simulink model "Basic_DMT"  (R2014b)
settings: Solver=FixedStepDiscrete  SolverMode=SingleTasking  StartTime=0.0  StopTime=25e-6-14e-9*24  RelTol=1e-3
PreLoadFcn:
  | userName = getenv('UserName');
  | 
  | if strcmp(userName,'Tim')
  | cd C:\Users\Tim\Documents\GitHub\MA_1\Basic_DMT
  | else
  | cd C:\Users\Tim-UML\Documents\GitHub\MA_1\Basic_DMT
  | end
InitFcn:
  | userName = getenv('UserName');
  | 
  | if strcmp(userName,'Tim')
  | cd C:\Users\Tim\Documents\GitHub\MA_1\Basic_DMT
  | else
  | cd C:\Users\Tim-UML\Documents\GitHub\MA_1\Basic_DMT
  | end
values from neighbouring files (symbols this model uses):
  a0 = 0.21194908595403703    (= 0.211949085954)    [initScript.m]
  a1 = 0.576101828091926    (= 0.576101828092)    [initScript.m]
  a2 = a0    (= 0.211949085954)    [initScript.m]
  beta = 1    [initScript.m]
  bitPerSymb = 4    [initScript.m]
  chanDownFact = Tchan/SystemPeriod    [initScript.m]
  fftLen = 16    [initScript.m]
  fftLenActive = fftLenDMT    (= 32)    [initScript.m]
  fftLenDMT = 2*fftLen    (= 32)    [initScript.m]
  GI_Active = GI_LenDMT    (= 0)    [initScript.m]
  GI_Len = 0    [initScript.m]
  GI_LenDMT = 0    [initScript.m]
  M = log2(fftLen)    [initScript.m]
  sysgenSystemPeriod = 4e-9    (= 4e-09)    [initScript.m]
  SystemPeriod = 4e-9    (= 4e-09)    [initScript.m]
  upsampleFactor = 1    [initScript.m]
  usedSubCar = 14    [initScript.m]
undefined symbols (not defined in the file or in its folder): bitCount, get, modu_mode, Tb, Ts
libraries: xbsIndex_r4 x822, commdigbbndam3 x59, simulink x42, dspsigops x7, commrandsrc2 x6, dspbuff3 x4, dspxfrm3 x3, dspswit3 x2, commseqgen2 x1, dsparch4 x1, commutil2 x1, dspsnks4 x1
(part 6 of 10)

== system Basic_DMT/Sysgen_Modulation/16-QAM4 ==
  In1 : Inport
  BitBasher : xbsIndex_r4/BitBasher  bitexpr=|  display_expr=on  sr_1=b  arith_type1=Unsigned  bin_pt1=0  sr_2=c  arith_type2=Unsigned  bin_pt2=0  sr_3=3  arith_type3=Unsigned  bin_pt3=0  sr_4=4  arith_type4=Unsigned  bin_pt4=0  dbl_ovrd=off  block_type=bitbasher
      | b={a[3:2]}
      | c={a[1:0]}
  Constant1 : xbsIndex_r4/Constant  const=-3  gui_display_data_type=Fixed-point  arith_type=Signed (2's comp)  n_bits=bitCount  bin_pt=fracLen  preci_type=Single  exp_width=8  frac_width=24  explicit_period=on  period=Ts*usedSubCar* bitPerSymb  equ=P=C  opselect=C  inp2=PCIN>>17  opr=+  inp1=P  carry=CIN  dbl_ovrd=off  block_type=constant
  Constant2 : xbsIndex_r4/Constant  const=-1  gui_display_data_type=Fixed-point  arith_type=Signed (2's comp)  n_bits=bitCount  bin_pt=fracLen  preci_type=Single  exp_width=8  frac_width=24  explicit_period=on  period=Ts*usedSubCar* bitPerSymb  equ=P=C  opselect=C  inp2=PCIN>>17  opr=+  inp1=P  carry=CIN  dbl_ovrd=off  block_type=constant
  Constant3 : xbsIndex_r4/Constant  const=3  gui_display_data_type=Fixed-point  arith_type=Signed (2's comp)  n_bits=bitCount  bin_pt=fracLen  preci_type=Single  exp_width=8  frac_width=24  explicit_period=on  period=Ts*usedSubCar* bitPerSymb  equ=P=C  opselect=C  inp2=PCIN>>17  opr=+  inp1=P  carry=CIN  dbl_ovrd=off  block_type=constant
  Constant4 : xbsIndex_r4/Constant  const=1  gui_display_data_type=Fixed-point  arith_type=Signed (2's comp)  n_bits=bitCount  bin_pt=fracLen  preci_type=Single  exp_width=8  frac_width=24  explicit_period=on  period=Ts*usedSubCar* bitPerSymb  equ=P=C  opselect=C  inp2=PCIN>>17  opr=+  inp1=P  carry=CIN  dbl_ovrd=off  block_type=constant
  Constant5 : xbsIndex_r4/Constant  const=1  gui_display_data_type=Fixed-point  arith_type=Signed (2's comp)  n_bits=bitCount  bin_pt=fracLen  preci_type=Single  exp_width=8  frac_width=24  explicit_period=on  period=Ts*usedSubCar* bitPerSymb  equ=P=C  opselect=C  inp2=PCIN>>17  opr=+  inp1=P  carry=CIN  dbl_ovrd=off  block_type=constant
  Constant6 : xbsIndex_r4/Constant  const=-3  gui_display_data_type=Fixed-point  arith_type=Signed (2's comp)  n_bits=bitCount  bin_pt=fracLen  preci_type=Single  exp_width=8  frac_width=24  explicit_period=on  period=Ts*usedSubCar* bitPerSymb  equ=P=C  opselect=C  inp2=PCIN>>17  opr=+  inp1=P  carry=CIN  dbl_ovrd=off  block_type=constant
  Constant7 : xbsIndex_r4/Constant  const=-1  gui_display_data_type=Fixed-point  arith_type=Signed (2's comp)  n_bits=bitCount  bin_pt=fracLen  preci_type=Single  exp_width=8  frac_width=24  explicit_period=on  period=Ts*usedSubCar* bitPerSymb  equ=P=C  opselect=C  inp2=PCIN>>17  opr=+  inp1=P  carry=CIN  dbl_ovrd=off  block_type=constant
  Constant9 : xbsIndex_r4/Constant  const=3  gui_display_data_type=Fixed-point  arith_type=Signed (2's comp)  n_bits=bitCount  bin_pt=fracLen  preci_type=Single  exp_width=8  frac_width=24  explicit_period=on  period=Ts*usedSubCar* bitPerSymb  equ=P=C  opselect=C  inp2=PCIN>>17  opr=+  inp1=P  carry=CIN  dbl_ovrd=off  block_type=constant
  Mux : xbsIndex_r4/Mux  inputs=4  en=off  latency=1  precision=Full  arith_type=Unsigned  n_bits=16  bin_pt=14  quantization=Truncate  overflow=Wrap  dbl_ovrd=off  block_type=mux
  Mux1 : xbsIndex_r4/Mux  inputs=4  en=off  latency=1  precision=Full  arith_type=Unsigned  n_bits=16  bin_pt=14  quantization=Truncate  overflow=Wrap  dbl_ovrd=off  block_type=mux
  Out2 : Outport
  Out3 : Outport  Port=2
  wires:
  Mux1/1 -> Out3/1
  In1/1 -> BitBasher/1
  Constant1/1 -> Mux/2
  Constant2/1 -> Mux/3
  BitBasher/1 -> Mux/1
  Constant9/1 -> Mux1/2
  Constant5/1 -> Mux1/3
  Constant7/1 -> Mux1/5
  Constant6/1 -> Mux1/4
  BitBasher/2 -> Mux1/1
  Constant4/1 -> Mux/5
  Mux/1 -> Out2/1
  Constant3/1 -> Mux/4

== system Basic_DMT/Sysgen_Modulation/16-QAM5 ==
  In1 : Inport
  BitBasher : xbsIndex_r4/BitBasher  bitexpr=|  display_expr=on  sr_1=b  arith_type1=Unsigned  bin_pt1=0  sr_2=c  arith_type2=Unsigned  bin_pt2=0  sr_3=3  arith_type3=Unsigned  bin_pt3=0  sr_4=4  arith_type4=Unsigned  bin_pt4=0  dbl_ovrd=off  block_type=bitbasher
      | b={a[3:2]}
      | c={a[1:0]}
  Constant1 : xbsIndex_r4/Constant  const=-3  gui_display_data_type=Fixed-point  arith_type=Signed (2's comp)  n_bits=bitCount  bin_pt=fracLen  preci_type=Single  exp_width=8  frac_width=24  explicit_period=on  period=Ts*usedSubCar* bitPerSymb  equ=P=C  opselect=C  inp2=PCIN>>17  opr=+  inp1=P  carry=CIN  dbl_ovrd=off  block_type=constant
  Constant2 : xbsIndex_r4/Constant  const=-1  gui_display_data_type=Fixed-point  arith_type=Signed (2's comp)  n_bits=bitCount  bin_pt=fracLen  preci_type=Single  exp_width=8  frac_width=24  explicit_period=on  period=Ts*usedSubCar* bitPerSymb  equ=P=C  opselect=C  inp2=PCIN>>17  opr=+  inp1=P  carry=CIN  dbl_ovrd=off  block_type=constant
  Constant3 : xbsIndex_r4/Constant  const=3  gui_display_data_type=Fixed-point  arith_type=Signed (2's comp)  n_bits=bitCount  bin_pt=fracLen  preci_type=Single  exp_width=8  frac_width=24  explicit_period=on  period=Ts*usedSubCar* bitPerSymb  equ=P=C  opselect=C  inp2=PCIN>>17  opr=+  inp1=P  carry=CIN  dbl_ovrd=off  block_type=constant
  Constant4 : xbsIndex_r4/Constant  const=1  gui_display_data_type=Fixed-point  arith_type=Signed (2's comp)  n_bits=bitCount  bin_pt=fracLen  preci_type=Single  exp_width=8  frac_width=24  explicit_period=on  period=Ts*usedSubCar* bitPerSymb  equ=P=C  opselect=C  inp2=PCIN>>17  opr=+  inp1=P  carry=CIN  dbl_ovrd=off  block_type=constant
  Constant5 : xbsIndex_r4/Constant  const=1  gui_display_data_type=Fixed-point  arith_type=Signed (2's comp)  n_bits=bitCount  bin_pt=fracLen  preci_type=Single  exp_width=8  frac_width=24  explicit_period=on  period=Ts*usedSubCar* bitPerSymb  equ=P=C  opselect=C  inp2=PCIN>>17  opr=+  inp1=P  carry=CIN  dbl_ovrd=off  block_type=constant
  Constant6 : xbsIndex_r4/Constant  const=-3  gui_display_data_type=Fixed-point  arith_type=Signed (2's comp)  n_bits=bitCount  bin_pt=fracLen  preci_type=Single  exp_width=8  frac_width=24  explicit_period=on  period=Ts*usedSubCar* bitPerSymb  equ=P=C  opselect=C  inp2=PCIN>>17  opr=+  inp1=P  carry=CIN  dbl_ovrd=off  block_type=constant
  Constant7 : xbsIndex_r4/Constant  const=-1  gui_display_data_type=Fixed-point  arith_type=Signed (2's comp)  n_bits=bitCount  bin_pt=fracLen  preci_type=Single  exp_width=8  frac_width=24  explicit_period=on  period=Ts*usedSubCar* bitPerSymb  equ=P=C  opselect=C  inp2=PCIN>>17  opr=+  inp1=P  carry=CIN  dbl_ovrd=off  block_type=constant
  Constant9 : xbsIndex_r4/Constant  const=3  gui_display_data_type=Fixed-point  arith_type=Signed (2's comp)  n_bits=bitCount  bin_pt=fracLen  preci_type=Single  exp_width=8  frac_width=24  explicit_period=on  period=Ts*usedSubCar* bitPerSymb  equ=P=C  opselect=C  inp2=PCIN>>17  opr=+  inp1=P  carry=CIN  dbl_ovrd=off  block_type=constant
  Mux : xbsIndex_r4/Mux  inputs=4  en=off  latency=1  precision=Full  arith_type=Unsigned  n_bits=16  bin_pt=14  quantization=Truncate  overflow=Wrap  dbl_ovrd=off  block_type=mux
  Mux1 : xbsIndex_r4/Mux  inputs=4  en=off  latency=1  precision=Full  arith_type=Unsigned  n_bits=16  bin_pt=14  quantization=Truncate  overflow=Wrap  dbl_ovrd=off  block_type=mux
  Out2 : Outport
  Out3 : Outport  Port=2
  wires:
  Mux1/1 -> Out3/1
  In1/1 -> BitBasher/1
  Constant1/1 -> Mux/2
  Constant2/1 -> Mux/3
  BitBasher/1 -> Mux/1
  Constant9/1 -> Mux1/2
  Constant5/1 -> Mux1/3
  Constant7/1 -> Mux1/5
  Constant6/1 -> Mux1/4
  BitBasher/2 -> Mux1/1
  Constant4/1 -> Mux/5
  Mux/1 -> Out2/1
  Constant3/1 -> Mux/4

== system Basic_DMT/Sysgen_Modulation/16-QAM6 ==
  In1 : Inport
  BitBasher : xbsIndex_r4/BitBasher  bitexpr=|  display_expr=on  sr_1=b  arith_type1=Unsigned  bin_pt1=0  sr_2=c  arith_type2=Unsigned  bin_pt2=0  sr_3=3  arith_type3=Unsigned  bin_pt3=0  sr_4=4  arith_type4=Unsigned  bin_pt4=0  dbl_ovrd=off  block_type=bitbasher
      | b={a[3:2]}
      | c={a[1:0]}
  Constant1 : xbsIndex_r4/Constant  const=-3  gui_display_data_type=Fixed-point  arith_type=Signed (2's comp)  n_bits=bitCount  bin_pt=fracLen  preci_type=Single  exp_width=8  frac_width=24  explicit_period=on  period=Ts*usedSubCar* bitPerSymb  equ=P=C  opselect=C  inp2=PCIN>>17  opr=+  inp1=P  carry=CIN  dbl_ovrd=off  block_type=constant
  Constant2 : xbsIndex_r4/Constant  const=-1  gui_display_data_type=Fixed-point  arith_type=Signed (2's comp)  n_bits=bitCount  bin_pt=fracLen  preci_type=Single  exp_width=8  frac_width=24  explicit_period=on  period=Ts*usedSubCar* bitPerSymb  equ=P=C  opselect=C  inp2=PCIN>>17  opr=+  inp1=P  carry=CIN  dbl_ovrd=off  block_type=constant
  Constant3 : xbsIndex_r4/Constant  const=3  gui_display_data_type=Fixed-point  arith_type=Signed (2's comp)  n_bits=bitCount  bin_pt=fracLen  preci_type=Single  exp_width=8  frac_width=24  explicit_period=on  period=Ts*usedSubCar* bitPerSymb  equ=P=C  opselect=C  inp2=PCIN>>17  opr=+  inp1=P  carry=CIN  dbl_ovrd=off  block_type=constant
  Constant4 : xbsIndex_r4/Constant  const=1  gui_display_data_type=Fixed-point  arith_type=Signed (2's comp)  n_bits=bitCount  bin_pt=fracLen  preci_type=Single  exp_width=8  frac_width=24  explicit_period=on  period=Ts*usedSubCar* bitPerSymb  equ=P=C  opselect=C  inp2=PCIN>>17  opr=+  inp1=P  carry=CIN  dbl_ovrd=off  block_type=constant
  Constant5 : xbsIndex_r4/Constant  const=1  gui_display_data_type=Fixed-point  arith_type=Signed (2's comp)  n_bits=bitCount  bin_pt=fracLen  preci_type=Single  exp_width=8  frac_width=24  explicit_period=on  period=Ts*usedSubCar* bitPerSymb  equ=P=C  opselect=C  inp2=PCIN>>17  opr=+  inp1=P  carry=CIN  dbl_ovrd=off  block_type=constant
  Constant6 : xbsIndex_r4/Constant  const=-3  gui_display_data_type=Fixed-point  arith_type=Signed (2's comp)  n_bits=bitCount  bin_pt=fracLen  preci_type=Single  exp_width=8  frac_width=24  explicit_period=on  period=Ts*usedSubCar* bitPerSymb  equ=P=C  opselect=C  inp2=PCIN>>17  opr=+  inp1=P  carry=CIN  dbl_ovrd=off  block_type=constant
  Constant7 : xbsIndex_r4/Constant  const=-1  gui_display_data_type=Fixed-point  arith_type=Signed (2's comp)  n_bits=bitCount  bin_pt=fracLen  preci_type=Single  exp_width=8  frac_width=24  explicit_period=on  period=Ts*usedSubCar* bitPerSymb  equ=P=C  opselect=C  inp2=PCIN>>17  opr=+  inp1=P  carry=CIN  dbl_ovrd=off  block_type=constant
  Constant9 : xbsIndex_r4/Constant  const=3  gui_display_data_type=Fixed-point  arith_type=Signed (2's comp)  n_bits=bitCount  bin_pt=fracLen  preci_type=Single  exp_width=8  frac_width=24  explicit_period=on  period=Ts*usedSubCar* bitPerSymb  equ=P=C  opselect=C  inp2=PCIN>>17  opr=+  inp1=P  carry=CIN  dbl_ovrd=off  block_type=constant
  Mux : xbsIndex_r4/Mux  inputs=4  en=off  latency=1  precision=Full  arith_type=Unsigned  n_bits=16  bin_pt=14  quantization=Truncate  overflow=Wrap  dbl_ovrd=off  block_type=mux
  Mux1 : xbsIndex_r4/Mux  inputs=4  en=off  latency=1  precision=Full  arith_type=Unsigned  n_bits=16  bin_pt=14  quantization=Truncate  overflow=Wrap  dbl_ovrd=off  block_type=mux
  Out2 : Outport
  Out3 : Outport  Port=2
  wires:
  Mux1/1 -> Out3/1
  In1/1 -> BitBasher/1
  Constant1/1 -> Mux/2
  Constant2/1 -> Mux/3
  BitBasher/1 -> Mux/1
  Constant9/1 -> Mux1/2
  Constant5/1 -> Mux1/3
  Constant7/1 -> Mux1/5
  Constant6/1 -> Mux1/4
  BitBasher/2 -> Mux1/1
  Constant4/1 -> Mux/5
  Mux/1 -> Out2/1
  Constant3/1 -> Mux/4

== system Basic_DMT/Sysgen_Modulation/16-QAM7 ==
  In1 : Inport
  BitBasher : xbsIndex_r4/BitBasher  bitexpr=|  display_expr=on  sr_1=b  arith_type1=Unsigned  bin_pt1=0  sr_2=c  arith_type2=Unsigned  bin_pt2=0  sr_3=3  arith_type3=Unsigned  bin_pt3=0  sr_4=4  arith_type4=Unsigned  bin_pt4=0  dbl_ovrd=off  block_type=bitbasher
      | b={a[3:2]}
      | c={a[1:0]}
  Constant1 : xbsIndex_r4/Constant  const=-3  gui_display_data_type=Fixed-point  arith_type=Signed (2's comp)  n_bits=bitCount  bin_pt=fracLen  preci_type=Single  exp_width=8  frac_width=24  explicit_period=on  period=Ts*usedSubCar* bitPerSymb  equ=P=C  opselect=C  inp2=PCIN>>17  opr=+  inp1=P  carry=CIN  dbl_ovrd=off  block_type=constant
  Constant2 : xbsIndex_r4/Constant  const=-1  gui_display_data_type=Fixed-point  arith_type=Signed (2's comp)  n_bits=bitCount  bin_pt=fracLen  preci_type=Single  exp_width=8  frac_width=24  explicit_period=on  period=Ts*usedSubCar* bitPerSymb  equ=P=C  opselect=C  inp2=PCIN>>17  opr=+  inp1=P  carry=CIN  dbl_ovrd=off  block_type=constant
  Constant3 : xbsIndex_r4/Constant  const=3  gui_display_data_type=Fixed-point  arith_type=Signed (2's comp)  n_bits=bitCount  bin_pt=fracLen  preci_type=Single  exp_width=8  frac_width=24  explicit_period=on  period=Ts*usedSubCar* bitPerSymb  equ=P=C  opselect=C  inp2=PCIN>>17  opr=+  inp1=P  carry=CIN  dbl_ovrd=off  block_type=constant
  Constant4 : xbsIndex_r4/Constant  const=1  gui_display_data_type=Fixed-point  arith_type=Signed (2's comp)  n_bits=bitCount  bin_pt=fracLen  preci_type=Single  exp_width=8  frac_width=24  explicit_period=on  period=Ts*usedSubCar* bitPerSymb  equ=P=C  opselect=C  inp2=PCIN>>17  opr=+  inp1=P  carry=CIN  dbl_ovrd=off  block_type=constant
  Constant5 : xbsIndex_r4/Constant  const=1  gui_display_data_type=Fixed-point  arith_type=Signed (2's comp)  n_bits=bitCount  bin_pt=fracLen  preci_type=Single  exp_width=8  frac_width=24  explicit_period=on  period=Ts*usedSubCar* bitPerSymb  equ=P=C  opselect=C  inp2=PCIN>>17  opr=+  inp1=P  carry=CIN  dbl_ovrd=off  block_type=constant
  Constant6 : xbsIndex_r4/Constant  const=-3  gui_display_data_type=Fixed-point  arith_type=Signed (2's comp)  n_bits=bitCount  bin_pt=fracLen  preci_type=Single  exp_width=8  frac_width=24  explicit_period=on  period=Ts*usedSubCar* bitPerSymb  equ=P=C  opselect=C  inp2=PCIN>>17  opr=+  inp1=P  carry=CIN  dbl_ovrd=off  block_type=constant
  Constant7 : xbsIndex_r4/Constant  const=-1  gui_display_data_type=Fixed-point  arith_type=Signed (2's comp)  n_bits=bitCount  bin_pt=fracLen  preci_type=Single  exp_width=8  frac_width=24  explicit_period=on  period=Ts*usedSubCar* bitPerSymb  equ=P=C  opselect=C  inp2=PCIN>>17  opr=+  inp1=P  carry=CIN  dbl_ovrd=off  block_type=constant
  Constant9 : xbsIndex_r4/Constant  const=3  gui_display_data_type=Fixed-point  arith_type=Signed (2's comp)  n_bits=bitCount  bin_pt=fracLen  preci_type=Single  exp_width=8  frac_width=24  explicit_period=on  period=Ts*usedSubCar* bitPerSymb  equ=P=C  opselect=C  inp2=PCIN>>17  opr=+  inp1=P  carry=CIN  dbl_ovrd=off  block_type=constant
  Mux : xbsIndex_r4/Mux  inputs=4  en=off  latency=1  precision=Full  arith_type=Unsigned  n_bits=16  bin_pt=14  quantization=Truncate  overflow=Wrap  dbl_ovrd=off  block_type=mux
  Mux1 : xbsIndex_r4/Mux  inputs=4  en=off  latency=1  precision=Full  arith_type=Unsigned  n_bits=16  bin_pt=14  quantization=Truncate  overflow=Wrap  dbl_ovrd=off  block_type=mux
  Out2 : Outport
  Out3 : Outport  Port=2
  wires:
  Mux1/1 -> Out3/1
  In1/1 -> BitBasher/1
  Constant1/1 -> Mux/2
  Constant2/1 -> Mux/3
  BitBasher/1 -> Mux/1
  Constant9/1 -> Mux1/2
  Constant5/1 -> Mux1/3
  Constant7/1 -> Mux1/5
  Constant6/1 -> Mux1/4
  BitBasher/2 -> Mux1/1
  Constant4/1 -> Mux/5
  Mux/1 -> Out2/1
  Constant3/1 -> Mux/4

== system Basic_DMT/Sysgen_Modulation/16-QAM8 ==
  In1 : Inport
  BitBasher : xbsIndex_r4/BitBasher  bitexpr=|  display_expr=on  sr_1=b  arith_type1=Unsigned  bin_pt1=0  sr_2=c  arith_type2=Unsigned  bin_pt2=0  sr_3=3  arith_type3=Unsigned  bin_pt3=0  sr_4=4  arith_type4=Unsigned  bin_pt4=0  dbl_ovrd=off  block_type=bitbasher
      | b={a[3:2]}
      | c={a[1:0]}
  Constant1 : xbsIndex_r4/Constant  const=-3  gui_display_data_type=Fixed-point  arith_type=Signed (2's comp)  n_bits=bitCount  bin_pt=fracLen  preci_type=Single  exp_width=8  frac_width=24  explicit_period=on  period=Ts*usedSubCar* bitPerSymb  equ=P=C  opselect=C  inp2=PCIN>>17  opr=+  inp1=P  carry=CIN  dbl_ovrd=off  block_type=constant
  Constant2 : xbsIndex_r4/Constant  const=-1  gui_display_data_type=Fixed-point  arith_type=Signed (2's comp)  n_bits=bitCount  bin_pt=fracLen  preci_type=Single  exp_width=8  frac_width=24  explicit_period=on  period=Ts*usedSubCar* bitPerSymb  equ=P=C  opselect=C  inp2=PCIN>>17  opr=+  inp1=P  carry=CIN  dbl_ovrd=off  block_type=constant
  Constant3 : xbsIndex_r4/Constant  const=3  gui_display_data_type=Fixed-point  arith_type=Signed (2's comp)  n_bits=bitCount  bin_pt=fracLen  preci_type=Single  exp_width=8  frac_width=24  explicit_period=on  period=Ts*usedSubCar* bitPerSymb  equ=P=C  opselect=C  inp2=PCIN>>17  opr=+  inp1=P  carry=CIN  dbl_ovrd=off  block_type=constant
  Constant4 : xbsIndex_r4/Constant  const=1  gui_display_data_type=Fixed-point  arith_type=Signed (2's comp)  n_bits=bitCount  bin_pt=fracLen  preci_type=Single  exp_width=8  frac_width=24  explicit_period=on  period=Ts*usedSubCar* bitPerSymb  equ=P=C  opselect=C  inp2=PCIN>>17  opr=+  inp1=P  carry=CIN  dbl_ovrd=off  block_type=constant
  Constant5 : xbsIndex_r4/Constant  const=1  gui_display_data_type=Fixed-point  arith_type=Signed (2's comp)  n_bits=bitCount  bin_pt=fracLen  preci_type=Single  exp_width=8  frac_width=24  explicit_period=on  period=Ts*usedSubCar* bitPerSymb  equ=P=C  opselect=C  inp2=PCIN>>17  opr=+  inp1=P  carry=CIN  dbl_ovrd=off  block_type=constant
  Constant6 : xbsIndex_r4/Constant  const=-3  gui_display_data_type=Fixed-point  arith_type=Signed (2's comp)  n_bits=bitCount  bin_pt=fracLen  preci_type=Single  exp_width=8  frac_width=24  explicit_period=on  period=Ts*usedSubCar* bitPerSymb  equ=P=C  opselect=C  inp2=PCIN>>17  opr=+  inp1=P  carry=CIN  dbl_ovrd=off  block_type=constant
  Constant7 : xbsIndex_r4/Constant  const=-1  gui_display_data_type=Fixed-point  arith_type=Signed (2's comp)  n_bits=bitCount  bin_pt=fracLen  preci_type=Single  exp_width=8  frac_width=24  explicit_period=on  period=Ts*usedSubCar* bitPerSymb  equ=P=C  opselect=C  inp2=PCIN>>17  opr=+  inp1=P  carry=CIN  dbl_ovrd=off  block_type=constant
  Constant9 : xbsIndex_r4/Constant  const=3  gui_display_data_type=Fixed-point  arith_type=Signed (2's comp)  n_bits=bitCount  bin_pt=fracLen  preci_type=Single  exp_width=8  frac_width=24  explicit_period=on  period=Ts*usedSubCar* bitPerSymb  equ=P=C  opselect=C  inp2=PCIN>>17  opr=+  inp1=P  carry=CIN  dbl_ovrd=off  block_type=constant
  Mux : xbsIndex_r4/Mux  inputs=4  en=off  latency=1  precision=Full  arith_type=Unsigned  n_bits=16  bin_pt=14  quantization=Truncate  overflow=Wrap  dbl_ovrd=off  block_type=mux
  Mux1 : xbsIndex_r4/Mux  inputs=4  en=off  latency=1  precision=Full  arith_type=Unsigned  n_bits=16  bin_pt=14  quantization=Truncate  overflow=Wrap  dbl_ovrd=off  block_type=mux
  Out2 : Outport
  Out3 : Outport  Port=2
  wires:
  Mux1/1 -> Out3/1
  In1/1 -> BitBasher/1
  Constant1/1 -> Mux/2
  Constant2/1 -> Mux/3
  BitBasher/1 -> Mux/1
  Constant9/1 -> Mux1/2
  Constant5/1 -> Mux1/3
  Constant7/1 -> Mux1/5
  Constant6/1 -> Mux1/4
  BitBasher/2 -> Mux1/1
  Constant4/1 -> Mux/5
  Mux/1 -> Out2/1
  Constant3/1 -> Mux/4

== system Basic_DMT/Sysgen_Modulation/16-QAM9 ==
  In1 : Inport
  BitBasher : xbsIndex_r4/BitBasher  bitexpr=|  display_expr=on  sr_1=b  arith_type1=Unsigned  bin_pt1=0  sr_2=c  arith_type2=Unsigned  bin_pt2=0  sr_3=3  arith_type3=Unsigned  bin_pt3=0  sr_4=4  arith_type4=Unsigned  bin_pt4=0  dbl_ovrd=off  block_type=bitbasher
      | b={a[3:2]}
      | c={a[1:0]}
  Constant1 : xbsIndex_r4/Constant  const=-3  gui_display_data_type=Fixed-point  arith_type=Signed (2's comp)  n_bits=bitCount  bin_pt=fracLen  preci_type=Single  exp_width=8  frac_width=24  explicit_period=on  period=Ts*usedSubCar* bitPerSymb  equ=P=C  opselect=C  inp2=PCIN>>17  opr=+  inp1=P  carry=CIN  dbl_ovrd=off  block_type=constant
  Constant2 : xbsIndex_r4/Constant  const=-1  gui_display_data_type=Fixed-point  arith_type=Signed (2's comp)  n_bits=bitCount  bin_pt=fracLen  preci_type=Single  exp_width=8  frac_width=24  explicit_period=on  period=Ts*usedSubCar* bitPerSymb  equ=P=C  opselect=C  inp2=PCIN>>17  opr=+  inp1=P  carry=CIN  dbl_ovrd=off  block_type=constant
  Constant3 : xbsIndex_r4/Constant  const=3  gui_display_data_type=Fixed-point  arith_type=Signed (2's comp)  n_bits=bitCount  bin_pt=fracLen  preci_type=Single  exp_width=8  frac_width=24  explicit_period=on  period=Ts*usedSubCar* bitPerSymb  equ=P=C  opselect=C  inp2=PCIN>>17  opr=+  inp1=P  carry=CIN  dbl_ovrd=off  block_type=constant
  Constant4 : xbsIndex_r4/Constant  const=1  gui_display_data_type=Fixed-point  arith_type=Signed (2's comp)  n_bits=bitCount  bin_pt=fracLen  preci_type=Single  exp_width=8  frac_width=24  explicit_period=on  period=Ts*usedSubCar* bitPerSymb  equ=P=C  opselect=C  inp2=PCIN>>17  opr=+  inp1=P  carry=CIN  dbl_ovrd=off  block_type=constant
  Constant5 : xbsIndex_r4/Constant  const=1  gui_display_data_type=Fixed-point  arith_type=Signed (2's comp)  n_bits=bitCount  bin_pt=fracLen  preci_type=Single  exp_width=8  frac_width=24  explicit_period=on  period=Ts*usedSubCar* bitPerSymb  equ=P=C  opselect=C  inp2=PCIN>>17  opr=+  inp1=P  carry=CIN  dbl_ovrd=off  block_type=constant
  Constant6 : xbsIndex_r4/Constant  const=-3  gui_display_data_type=Fixed-point  arith_type=Signed (2's comp)  n_bits=bitCount  bin_pt=fracLen  preci_type=Single  exp_width=8  frac_width=24  explicit_period=on  period=Ts*usedSubCar* bitPerSymb  equ=P=C  opselect=C  inp2=PCIN>>17  opr=+  inp1=P  carry=CIN  dbl_ovrd=off  block_type=constant
  Constant7 : xbsIndex_r4/Constant  const=-1  gui_display_data_type=Fixed-point  arith_type=Signed (2's comp)  n_bits=bitCount  bin_pt=fracLen  preci_type=Single  exp_width=8  frac_width=24  explicit_period=on  period=Ts*usedSubCar* bitPerSymb  equ=P=C  opselect=C  inp2=PCIN>>17  opr=+  inp1=P  carry=CIN  dbl_ovrd=off  block_type=constant
  Constant9 : xbsIndex_r4/Constant  const=3  gui_display_data_type=Fixed-point  arith_type=Signed (2's comp)  n_bits=bitCount  bin_pt=fracLen  preci_type=Single  exp_width=8  frac_width=24  explicit_period=on  period=Ts*usedSubCar* bitPerSymb  equ=P=C  opselect=C  inp2=PCIN>>17  opr=+  inp1=P  carry=CIN  dbl_ovrd=off  block_type=constant
  Mux : xbsIndex_r4/Mux  inputs=4  en=off  latency=1  precision=Full  arith_type=Unsigned  n_bits=16  bin_pt=14  quantization=Truncate  overflow=Wrap  dbl_ovrd=off  block_type=mux
  Mux1 : xbsIndex_r4/Mux  inputs=4  en=off  latency=1  precision=Full  arith_type=Unsigned  n_bits=16  bin_pt=14  quantization=Truncate  overflow=Wrap  dbl_ovrd=off  block_type=mux
  Out2 : Outport
  Out3 : Outport  Port=2
  wires:
  Mux1/1 -> Out3/1
  In1/1 -> BitBasher/1
  Constant1/1 -> Mux/2
  Constant2/1 -> Mux/3
  BitBasher/1 -> Mux/1
  Constant9/1 -> Mux1/2
  Constant5/1 -> Mux1/3
  Constant7/1 -> Mux1/5
  Constant6/1 -> Mux1/4
  BitBasher/2 -> Mux1/1
  Constant4/1 -> Mux/5
  Mux/1 -> Out2/1
  Constant3/1 -> Mux/4

== system Basic_DMT/Sysgen_SIPaFFT/Delay_GI ==
  note: 1) Add Subsystem or Model blocks as valid variant choices.
      | 2) You cannot connect blocks at this level. At simulation, connectivity is automatically
      | determined, based on the active variant and port name matching.
  Inp_Re : Inport
  Inp_Im : Inport  Port=2
  GI_Delay_DMT : Subsystem  VariantControl=guardInterval==2&&dmtOfdm==2
  No_Delay : Subsystem  VariantControl=guardInterval==1||dmtOfdm==1
  Out_Re : Outport
  Out_Im : Outport  Port=2

== system Basic_DMT/Sysgen_SIPaFFT/Delay_Guard_Interval2 ==
  note: 1) Add Subsystem or Model blocks as valid variant choices.
      | 2) You cannot connect blocks at this level. At simulation, connectivity is automatically
      | determined, based on the active variant and port name matching.
  Re : Inport
  Im : Inport  Port=2
  No_equal : Subsystem  VariantControl=equalizer==1
  Yes_equal : Subsystem  VariantControl=equalizer==2
  Re_Sub1 : Outport
  Im_Sub1 : Outport  Port=2
  Re_Sub2 : Outport  Port=3
  Im_Sub2 : Outport  Port=4
  Re_Sub3 : Outport  Port=5
  Im_Sub3 : Outport  Port=6
  Re_Sub4 : Outport  Port=7
  Im_Sub4 : Outport  Port=8
  Re_Sub5 : Outport  Port=9
  Im_Sub5 : Outport  Port=10
  Re_Sub6 : Outport  Port=11
  Im_Sub6 : Outport  Port=12
  Re_Sub7 : Outport  Port=13
  Im_Sub7 : Outport  Port=14
  Re_Sub8 : Outport  Port=15
  Im_Sub8 : Outport  Port=16
  Re_Sub9 : Outport  Port=17
  Im_Sub9 : Outport  Port=18
  Re_Sub10 : Outport  Port=19
  Im_Sub10 : Outport  Port=20
  Re_Sub11 : Outport  Port=21
  Im_Sub11 : Outport  Port=22
  Re_Sub12 : Outport  Port=23
  Im_Sub12 : Outport  Port=24
  Re_Sub13 : Outport  Port=25
  Im_Sub13 : Outport  Port=26
  Re_Sub14 : Outport  Port=27
  Im_Sub14 : Outport  Port=28
  Re_Sub15 : Outport  Port=29
  Im_Sub15 : Outport  Port=30
  Re_Sub16 : Outport  Port=31
  Im_Sub16 : Outport  Port=32

== system Basic_DMT/Sysgen_SIPaFFT/FFT ==
  note: 1) Add Subsystem or Model blocks as valid variant choices.
      | 2) You cannot connect blocks at this level. At simulation, connectivity is automatically
      | determined, based on the active variant and port name matching.
  sg_Re : Inport
  sg_Im : Inport  Port=2
  FFT_DMT : Subsystem  VariantControl=dmtOfdm==2
  FFT_OFDM : Subsystem  VariantControl=dmtOfdm==1
  Re_out : Outport
  Im_out : Outport  Port=2
  db_aft_DMT_Re : Outport  Port=3
  db_aft_DMT_Im : Outport  Port=4

== system Basic_DMT/Sysgen_SIPaFFT/Guard_Interval ==
  note: 1) Add Subsystem or Model blocks as valid variant choices.
      | 2) You cannot connect blocks at this level. At simulation, connectivity is automatically
      | determined, based on the active variant and port name matching.
  Re_In : Inport
  Im_In : Inport  Port=2
  None : Subsystem  VariantControl=guardInterval==1
  Rem_GI_DMT : Subsystem  VariantControl=guardInterval==2&&dmtOfdm==2
  Rem_GI_OFDM : Subsystem  VariantControl=guardInterval==2&&dmtOfdm==1
  Re : Outport
  Im : Outport  Port=2

== system Basic_DMT/Channel/Yes_Channel/Delay_upsample ==
  note: 1) Add Subsystem or Model blocks as valid variant choices.
      | 2) You cannot connect blocks at this level. At simulation, connectivity is automatically
      | determined, based on the active variant and port name matching.
  In1 : Inport
  Del_ups : Subsystem  VariantControl=upsample==2
  Delay_None : Subsystem  VariantControl=upsample==1
  Out1 : Outport

== system Basic_DMT/Demodulation/Bit Demapping P1/16-QAM ==
  In1 : Inport
  Enable : EnablePort
  Rectangular QAM Demodulator Baseband : commdigbbndam3/Rectangular QAM Demodulator Baseband  M=16  PowType=Min. distance between symbols  MinDist=2  AvgPow=1  PeakPow=1  Ph=0  Dec=Gray  Mapping=[0:15]  OutType=Bit  DecType=Hard decision  VarSource=Dialog  Variance=1  outDtype1=boolean  outDtype2=Inherit via internal rule  derotateFactorWordLen=16  denormFactorWordLen=16  prodOutWordLen=32  prodOutRoundingMode=Convergent  prodOutOverflowMode=Saturate  sumWordLen=32
  Out1 : Outport
  wires:
  In1/1 -> Rectangular QAM Demodulator Baseband/1
  Rectangular QAM Demodulator Baseband/1 -> Out1/1

== system Basic_DMT/Demodulation/Bit Demapping P1/256-QAM ==
  In1 : Inport
  Enable : EnablePort
  Complex to Real-Imag : ComplexToRealImag  Commented=on
  Eye Diagram : EyeDiagram  Commented=on
  Rectangular QAM Demodulator Baseband : commdigbbndam3/Rectangular QAM Demodulator Baseband  M=16  PowType=Min. distance between symbols  MinDist=2  AvgPow=1  PeakPow=1  Ph=0  Dec=Gray  Mapping=[0:15]  OutType=Bit  DecType=Hard decision  VarSource=Dialog  Variance=1  outDtype1=boolean  outDtype2=Inherit via internal rule  derotateFactorWordLen=16  denormFactorWordLen=16  prodOutWordLen=32  prodOutRoundingMode=Convergent  prodOutOverflowMode=Saturate  sumWordLen=32
  Scope : Scope  Commented=on  NumInputPorts=2
      settings: YMin=-5~-5  YMax=5~5  SaveName=ScopeData44
  Out1 : Outport
  wires:
  Rectangular QAM Demodulator Baseband/1 -> Out1/1
  In1/1 -> Eye Diagram/1, Complex to Real-Imag/1, Rectangular QAM Demodulator Baseband/1
  Complex to Real-Imag/1 -> Scope/1
  Complex to Real-Imag/2 -> Scope/2

== system Basic_DMT/Demodulation/Bit Demapping P10/16-QAM ==
  In1 : Inport
  Enable : EnablePort
  Rectangular QAM Demodulator Baseband : commdigbbndam3/Rectangular QAM Demodulator Baseband  M=16  PowType=Min. distance between symbols  MinDist=2  AvgPow=1  PeakPow=1  Ph=0  Dec=Gray  Mapping=[0:15]  OutType=Bit  DecType=Hard decision  VarSource=Dialog  Variance=1  outDtype1=boolean  outDtype2=Inherit via internal rule  derotateFactorWordLen=16  denormFactorWordLen=16  prodOutWordLen=32  prodOutRoundingMode=Convergent  prodOutOverflowMode=Saturate  sumWordLen=32
  Out1 : Outport
  wires:
  In1/1 -> Rectangular QAM Demodulator Baseband/1
  Rectangular QAM Demodulator Baseband/1 -> Out1/1

== system Basic_DMT/Demodulation/Bit Demapping P10/256-QAM ==
  In1 : Inport
  Enable : EnablePort
  Rectangular QAM Demodulator Baseband : commdigbbndam3/Rectangular QAM Demodulator Baseband  M=16  PowType=Min. distance between symbols  MinDist=2  AvgPow=1  PeakPow=1  Ph=0  Dec=Gray  Mapping=[0:15]  OutType=Bit  DecType=Hard decision  VarSource=Dialog  Variance=1  outDtype1=boolean  outDtype2=Inherit via internal rule  derotateFactorWordLen=16  denormFactorWordLen=16  prodOutWordLen=32  prodOutRoundingMode=Convergent  prodOutOverflowMode=Saturate  sumWordLen=32
  Out1 : Outport
  wires:
  Rectangular QAM Demodulator Baseband/1 -> Out1/1
  In1/1 -> Rectangular QAM Demodulator Baseband/1

== system Basic_DMT/Demodulation/Bit Demapping P11/16-QAM ==
  In1 : Inport
  Enable : EnablePort
  Rectangular QAM Demodulator Baseband : commdigbbndam3/Rectangular QAM Demodulator Baseband  M=16  PowType=Min. distance between symbols  MinDist=2  AvgPow=1  PeakPow=1  Ph=0  Dec=Gray  Mapping=[0:15]  OutType=Bit  DecType=Hard decision  VarSource=Dialog  Variance=1  outDtype1=boolean  outDtype2=Inherit via internal rule  derotateFactorWordLen=16  denormFactorWordLen=16  prodOutWordLen=32  prodOutRoundingMode=Convergent  prodOutOverflowMode=Saturate  sumWordLen=32
  Out1 : Outport
  wires:
  In1/1 -> Rectangular QAM Demodulator Baseband/1
  Rectangular QAM Demodulator Baseband/1 -> Out1/1

== system Basic_DMT/Demodulation/Bit Demapping P11/256-QAM ==
  In1 : Inport
  Enable : EnablePort
  Rectangular QAM Demodulator Baseband : commdigbbndam3/Rectangular QAM Demodulator Baseband  M=16  PowType=Min. distance between symbols  MinDist=2  AvgPow=1  PeakPow=1  Ph=0  Dec=Gray  Mapping=[0:15]  OutType=Bit  DecType=Hard decision  VarSource=Dialog  Variance=1  outDtype1=boolean  outDtype2=Inherit via internal rule  derotateFactorWordLen=16  denormFactorWordLen=16  prodOutWordLen=32  prodOutRoundingMode=Convergent  prodOutOverflowMode=Saturate  sumWordLen=32
  Out1 : Outport
  wires:
  Rectangular QAM Demodulator Baseband/1 -> Out1/1
  In1/1 -> Rectangular QAM Demodulator Baseband/1

== system Basic_DMT/Demodulation/Bit Demapping P12/16-QAM ==
  In1 : Inport
  Enable : EnablePort
  Rectangular QAM Demodulator Baseband : commdigbbndam3/Rectangular QAM Demodulator Baseband  M=16  PowType=Min. distance between symbols  MinDist=2  AvgPow=1  PeakPow=1  Ph=0  Dec=Gray  Mapping=[0:15]  OutType=Bit  DecType=Hard decision  VarSource=Dialog  Variance=1  outDtype1=boolean  outDtype2=Inherit via internal rule  derotateFactorWordLen=16  denormFactorWordLen=16  prodOutWordLen=32  prodOutRoundingMode=Convergent  prodOutOverflowMode=Saturate  sumWordLen=32
  Out1 : Outport
  wires:
  In1/1 -> Rectangular QAM Demodulator Baseband/1
  Rectangular QAM Demodulator Baseband/1 -> Out1/1

== system Basic_DMT/Demodulation/Bit Demapping P12/256-QAM ==
  In1 : Inport
  Enable : EnablePort
  Rectangular QAM Demodulator Baseband : commdigbbndam3/Rectangular QAM Demodulator Baseband  M=16  PowType=Min. distance between symbols  MinDist=2  AvgPow=1  PeakPow=1  Ph=0  Dec=Gray  Mapping=[0:15]  OutType=Bit  DecType=Hard decision  VarSource=Dialog  Variance=1  outDtype1=boolean  outDtype2=Inherit via internal rule  derotateFactorWordLen=16  denormFactorWordLen=16  prodOutWordLen=32  prodOutRoundingMode=Convergent  prodOutOverflowMode=Saturate  sumWordLen=32
  Out1 : Outport
  wires:
  Rectangular QAM Demodulator Baseband/1 -> Out1/1
  In1/1 -> Rectangular QAM Demodulator Baseband/1

== system Basic_DMT/Demodulation/Bit Demapping P13/16-QAM ==
  In1 : Inport
  Enable : EnablePort
  Rectangular QAM Demodulator Baseband : commdigbbndam3/Rectangular QAM Demodulator Baseband  M=16  PowType=Min. distance between symbols  MinDist=2  AvgPow=1  PeakPow=1  Ph=0  Dec=Gray  Mapping=[0:15]  OutType=Bit  DecType=Hard decision  VarSource=Dialog  Variance=1  outDtype1=boolean  outDtype2=Inherit via internal rule  derotateFactorWordLen=16  denormFactorWordLen=16  prodOutWordLen=32  prodOutRoundingMode=Convergent  prodOutOverflowMode=Saturate  sumWordLen=32
  Out1 : Outport
  wires:
  In1/1 -> Rectangular QAM Demodulator Baseband/1
  Rectangular QAM Demodulator Baseband/1 -> Out1/1

== system Basic_DMT/Demodulation/Bit Demapping P13/256-QAM ==
  In1 : Inport
  Enable : EnablePort
  Rectangular QAM Demodulator Baseband : commdigbbndam3/Rectangular QAM Demodulator Baseband  M=16  PowType=Min. distance between symbols  MinDist=2  AvgPow=1  PeakPow=1  Ph=0  Dec=Gray  Mapping=[0:15]  OutType=Bit  DecType=Hard decision  VarSource=Dialog  Variance=1  outDtype1=boolean  outDtype2=Inherit via internal rule  derotateFactorWordLen=16  denormFactorWordLen=16  prodOutWordLen=32  prodOutRoundingMode=Convergent  prodOutOverflowMode=Saturate  sumWordLen=32
  Out1 : Outport
  wires:
  Rectangular QAM Demodulator Baseband/1 -> Out1/1
  In1/1 -> Rectangular QAM Demodulator Baseband/1

== system Basic_DMT/Demodulation/Bit Demapping P14/16-QAM ==
  In1 : Inport
  Enable : EnablePort
  Rectangular QAM Demodulator Baseband : commdigbbndam3/Rectangular QAM Demodulator Baseband  M=16  PowType=Min. distance between symbols  MinDist=2  AvgPow=1  PeakPow=1  Ph=0  Dec=Gray  Mapping=[0:15]  OutType=Bit  DecType=Hard decision  VarSource=Dialog  Variance=1  outDtype1=boolean  outDtype2=Inherit via internal rule  derotateFactorWordLen=16  denormFactorWordLen=16  prodOutWordLen=32  prodOutRoundingMode=Convergent  prodOutOverflowMode=Saturate  sumWordLen=32
  Out1 : Outport
  wires:
  In1/1 -> Rectangular QAM Demodulator Baseband/1
  Rectangular QAM Demodulator Baseband/1 -> Out1/1

== system Basic_DMT/Demodulation/Bit Demapping P14/256-QAM ==
  In1 : Inport
  Enable : EnablePort
  Rectangular QAM Demodulator Baseband : commdigbbndam3/Rectangular QAM Demodulator Baseband  M=16  PowType=Min. distance between symbols  MinDist=2  AvgPow=1  PeakPow=1  Ph=0  Dec=Gray  Mapping=[0:15]  OutType=Bit  DecType=Hard decision  VarSource=Dialog  Variance=1  outDtype1=boolean  outDtype2=Inherit via internal rule  derotateFactorWordLen=16  denormFactorWordLen=16  prodOutWordLen=32  prodOutRoundingMode=Convergent  prodOutOverflowMode=Saturate  sumWordLen=32
  Out1 : Outport
  wires:
  Rectangular QAM Demodulator Baseband/1 -> Out1/1
  In1/1 -> Rectangular QAM Demodulator Baseband/1

== system Basic_DMT/Demodulation/Bit Demapping P2/16-QAM ==
  In1 : Inport
  Enable : EnablePort
  Rectangular QAM Demodulator Baseband : commdigbbndam3/Rectangular QAM Demodulator Baseband  M=16  PowType=Min. distance between symbols  MinDist=2  AvgPow=1  PeakPow=1  Ph=0  Dec=Gray  Mapping=[0:15]  OutType=Bit  DecType=Hard decision  VarSource=Dialog  Variance=1  outDtype1=boolean  outDtype2=Inherit via internal rule  derotateFactorWordLen=16  denormFactorWordLen=16  prodOutWordLen=32  prodOutRoundingMode=Convergent  prodOutOverflowMode=Saturate  sumWordLen=32
  Out1 : Outport
  wires:
  In1/1 -> Rectangular QAM Demodulator Baseband/1
  Rectangular QAM Demodulator Baseband/1 -> Out1/1

== system Basic_DMT/Demodulation/Bit Demapping P2/256-QAM ==
  In1 : Inport
  Enable : EnablePort
  Rectangular QAM Demodulator Baseband : commdigbbndam3/Rectangular QAM Demodulator Baseband  M=16  PowType=Min. distance between symbols  MinDist=2  AvgPow=1  PeakPow=1  Ph=0  Dec=Gray  Mapping=[0:15]  OutType=Bit  DecType=Hard decision  VarSource=Dialog  Variance=1  outDtype1=boolean  outDtype2=Inherit via internal rule  derotateFactorWordLen=16  denormFactorWordLen=16  prodOutWordLen=32  prodOutRoundingMode=Convergent  prodOutOverflowMode=Saturate  sumWordLen=32
  Out1 : Outport
  wires:
  Rectangular QAM Demodulator Baseband/1 -> Out1/1
  In1/1 -> Rectangular QAM Demodulator Baseband/1

== system Basic_DMT/Demodulation/Bit Demapping P3/16-QAM ==
  In1 : Inport
  Enable : EnablePort
  Rectangular QAM Demodulator Baseband : commdigbbndam3/Rectangular QAM Demodulator Baseband  M=16  PowType=Min. distance between symbols  MinDist=2  AvgPow=1  PeakPow=1  Ph=0  Dec=Gray  Mapping=[0:15]  OutType=Bit  DecType=Hard decision  VarSource=Dialog  Variance=1  outDtype1=boolean  outDtype2=Inherit via internal rule  derotateFactorWordLen=16  denormFactorWordLen=16  prodOutWordLen=32  prodOutRoundingMode=Convergent  prodOutOverflowMode=Saturate  sumWordLen=32
  Out1 : Outport
  wires:
  In1/1 -> Rectangular QAM Demodulator Baseband/1
  Rectangular QAM Demodulator Baseband/1 -> Out1/1

== system Basic_DMT/Demodulation/Bit Demapping P3/256-QAM ==
  In1 : Inport
  Enable : EnablePort
  Rectangular QAM Demodulator Baseband : commdigbbndam3/Rectangular QAM Demodulator Baseband  M=16  PowType=Min. distance between symbols  MinDist=2  AvgPow=1  PeakPow=1  Ph=0  Dec=Gray  Mapping=[0:15]  OutType=Bit  DecType=Hard decision  VarSource=Dialog  Variance=1  outDtype1=boolean  outDtype2=Inherit via internal rule  derotateFactorWordLen=16  denormFactorWordLen=16  prodOutWordLen=32  prodOutRoundingMode=Convergent  prodOutOverflowMode=Saturate  sumWordLen=32
  Out1 : Outport
  wires:
  Rectangular QAM Demodulator Baseband/1 -> Out1/1
  In1/1 -> Rectangular QAM Demodulator Baseband/1

== system Basic_DMT/Demodulation/Bit Demapping P4/16-QAM ==
  In1 : Inport
  Enable : EnablePort
  Rectangular QAM Demodulator Baseband : commdigbbndam3/Rectangular QAM Demodulator Baseband  M=16  PowType=Min. distance between symbols  MinDist=2  AvgPow=1  PeakPow=1  Ph=0  Dec=Gray  Mapping=[0:15]  OutType=Bit  DecType=Hard decision  VarSource=Dialog  Variance=1  outDtype1=boolean  outDtype2=Inherit via internal rule  derotateFactorWordLen=16  denormFactorWordLen=16  prodOutWordLen=32  prodOutRoundingMode=Convergent  prodOutOverflowMode=Saturate  sumWordLen=32
  Out1 : Outport
  wires:
  In1/1 -> Rectangular QAM Demodulator Baseband/1
  Rectangular QAM Demodulator Baseband/1 -> Out1/1

== system Basic_DMT/Demodulation/Bit Demapping P4/256-QAM ==
  In1 : Inport
  Enable : EnablePort
  Rectangular QAM Demodulator Baseband : commdigbbndam3/Rectangular QAM Demodulator Baseband  M=16  PowType=Min. distance between symbols  MinDist=2  AvgPow=1  PeakPow=1  Ph=0  Dec=Gray  Mapping=[0:15]  OutType=Bit  DecType=Hard decision  VarSource=Dialog  Variance=1  outDtype1=boolean  outDtype2=Inherit via internal rule  derotateFactorWordLen=16  denormFactorWordLen=16  prodOutWordLen=32  prodOutRoundingMode=Convergent  prodOutOverflowMode=Saturate  sumWordLen=32
  Out1 : Outport
  wires:
  Rectangular QAM Demodulator Baseband/1 -> Out1/1
  In1/1 -> Rectangular QAM Demodulator Baseband/1

== system Basic_DMT/Demodulation/Bit Demapping P5/16-QAM ==
  In1 : Inport
  Enable : EnablePort
  Rectangular QAM Demodulator Baseband : commdigbbndam3/Rectangular QAM Demodulator Baseband  M=16  PowType=Min. distance between symbols  MinDist=2  AvgPow=1  PeakPow=1  Ph=0  Dec=Gray  Mapping=[0:15]  OutType=Bit  DecType=Hard decision  VarSource=Dialog  Variance=1  outDtype1=boolean  outDtype2=Inherit via internal rule  derotateFactorWordLen=16  denormFactorWordLen=16  prodOutWordLen=32  prodOutRoundingMode=Convergent  prodOutOverflowMode=Saturate  sumWordLen=32
  Out1 : Outport
  wires:
  In1/1 -> Rectangular QAM Demodulator Baseband/1
  Rectangular QAM Demodulator Baseband/1 -> Out1/1

== system Basic_DMT/Demodulation/Bit Demapping P5/256-QAM ==
  In1 : Inport
  Enable : EnablePort
  Rectangular QAM Demodulator Baseband : commdigbbndam3/Rectangular QAM Demodulator Baseband  M=16  PowType=Min. distance between symbols  MinDist=2  AvgPow=1  PeakPow=1  Ph=0  Dec=Gray  Mapping=[0:15]  OutType=Bit  DecType=Hard decision  VarSource=Dialog  Variance=1  outDtype1=boolean  outDtype2=Inherit via internal rule  derotateFactorWordLen=16  denormFactorWordLen=16  prodOutWordLen=32  prodOutRoundingMode=Convergent  prodOutOverflowMode=Saturate  sumWordLen=32
  Out1 : Outport
  wires:
  Rectangular QAM Demodulator Baseband/1 -> Out1/1
  In1/1 -> Rectangular QAM Demodulator Baseband/1

== system Basic_DMT/Demodulation/Bit Demapping P6/16-QAM ==
  In1 : Inport
  Enable : EnablePort
  Rectangular QAM Demodulator Baseband : commdigbbndam3/Rectangular QAM Demodulator Baseband  M=16  PowType=Min. distance between symbols  MinDist=2  AvgPow=1  PeakPow=1  Ph=0  Dec=Gray  Mapping=[0:15]  OutType=Bit  DecType=Hard decision  VarSource=Dialog  Variance=1  outDtype1=boolean  outDtype2=Inherit via internal rule  derotateFactorWordLen=16  denormFactorWordLen=16  prodOutWordLen=32  prodOutRoundingMode=Convergent  prodOutOverflowMode=Saturate  sumWordLen=32
  Out1 : Outport
  wires:
  In1/1 -> Rectangular QAM Demodulator Baseband/1
  Rectangular QAM Demodulator Baseband/1 -> Out1/1

== system Basic_DMT/Demodulation/Bit Demapping P6/256-QAM ==
  In1 : Inport
  Enable : EnablePort
  Rectangular QAM Demodulator Baseband : commdigbbndam3/Rectangular QAM Demodulator Baseband  M=16  PowType=Min. distance between symbols  MinDist=2  AvgPow=1  PeakPow=1  Ph=0  Dec=Gray  Mapping=[0:15]  OutType=Bit  DecType=Hard decision  VarSource=Dialog  Variance=1  outDtype1=boolean  outDtype2=Inherit via internal rule  derotateFactorWordLen=16  denormFactorWordLen=16  prodOutWordLen=32  prodOutRoundingMode=Convergent  prodOutOverflowMode=Saturate  sumWordLen=32
  Out1 : Outport
  wires:
  Rectangular QAM Demodulator Baseband/1 -> Out1/1
  In1/1 -> Rectangular QAM Demodulator Baseband/1

== system Basic_DMT/Demodulation/Bit Demapping P7/16-QAM ==
  In1 : Inport
  Enable : EnablePort
  Rectangular QAM Demodulator Baseband : commdigbbndam3/Rectangular QAM Demodulator Baseband  M=16  PowType=Min. distance between symbols  MinDist=2  AvgPow=1  PeakPow=1  Ph=0  Dec=Gray  Mapping=[0:15]  OutType=Bit  DecType=Hard decision  VarSource=Dialog  Variance=1  outDtype1=boolean  outDtype2=Inherit via internal rule  derotateFactorWordLen=16  denormFactorWordLen=16  prodOutWordLen=32  prodOutRoundingMode=Convergent  prodOutOverflowMode=Saturate  sumWordLen=32
  Out1 : Outport
  wires:
  In1/1 -> Rectangular QAM Demodulator Baseband/1
  Rectangular QAM Demodulator Baseband/1 -> Out1/1

== system Basic_DMT/Demodulation/Bit Demapping P7/256-QAM ==
  In1 : Inport
  Enable : EnablePort
  Rectangular QAM Demodulator Baseband : commdigbbndam3/Rectangular QAM Demodulator Baseband  M=16  PowType=Min. distance between symbols  MinDist=2  AvgPow=1  PeakPow=1  Ph=0  Dec=Gray  Mapping=[0:15]  OutType=Bit  DecType=Hard decision  VarSource=Dialog  Variance=1  outDtype1=boolean  outDtype2=Inherit via internal rule  derotateFactorWordLen=16  denormFactorWordLen=16  prodOutWordLen=32  prodOutRoundingMode=Convergent  prodOutOverflowMode=Saturate  sumWordLen=32
  Out1 : Outport
  wires:
  Rectangular QAM Demodulator Baseband/1 -> Out1/1
  In1/1 -> Rectangular QAM Demodulator Baseband/1

== system Basic_DMT/Demodulation/Bit Demapping P8/16-QAM ==
  In1 : Inport
  Enable : EnablePort
  Rectangular QAM Demodulator Baseband : commdigbbndam3/Rectangular QAM Demodulator Baseband  M=16  PowType=Min. distance between symbols  MinDist=2  AvgPow=1  PeakPow=1  Ph=0  Dec=Gray  Mapping=[0:15]  OutType=Bit  DecType=Hard decision  VarSource=Dialog  Variance=1  outDtype1=boolean  outDtype2=Inherit via internal rule  derotateFactorWordLen=16  denormFactorWordLen=16  prodOutWordLen=32  prodOutRoundingMode=Convergent  prodOutOverflowMode=Saturate  sumWordLen=32
  Out1 : Outport
  wires:
  In1/1 -> Rectangular QAM Demodulator Baseband/1
  Rectangular QAM Demodulator Baseband/1 -> Out1/1

== system Basic_DMT/Demodulation/Bit Demapping P8/256-QAM ==
  In1 : Inport
  Enable : EnablePort
  Rectangular QAM Demodulator Baseband : commdigbbndam3/Rectangular QAM Demodulator Baseband  M=16  PowType=Min. distance between symbols  MinDist=2  AvgPow=1  PeakPow=1  Ph=0  Dec=Gray  Mapping=[0:15]  OutType=Bit  DecType=Hard decision  VarSource=Dialog  Variance=1  outDtype1=boolean  outDtype2=Inherit via internal rule  derotateFactorWordLen=16  denormFactorWordLen=16  prodOutWordLen=32  prodOutRoundingMode=Convergent  prodOutOverflowMode=Saturate  sumWordLen=32
  Out1 : Outport
  wires:
  Rectangular QAM Demodulator Baseband/1 -> Out1/1
  In1/1 -> Rectangular QAM Demodulator Baseband/1

== system Basic_DMT/Demodulation/Bit Demapping P9/16-QAM ==
  In1 : Inport
  Enable : EnablePort
  Rectangular QAM Demodulator Baseband : commdigbbndam3/Rectangular QAM Demodulator Baseband  M=16  PowType=Min. distance between symbols  MinDist=2  AvgPow=1  PeakPow=1  Ph=0  Dec=Gray  Mapping=[0:15]  OutType=Bit  DecType=Hard decision  VarSource=Dialog  Variance=1  outDtype1=boolean  outDtype2=Inherit via internal rule  derotateFactorWordLen=16  denormFactorWordLen=16  prodOutWordLen=32  prodOutRoundingMode=Convergent  prodOutOverflowMode=Saturate  sumWordLen=32
  Out1 : Outport
  wires:
  In1/1 -> Rectangular QAM Demodulator Baseband/1
  Rectangular QAM Demodulator Baseband/1 -> Out1/1

== system Basic_DMT/Demodulation/Bit Demapping P9/256-QAM ==
  In1 : Inport
  Enable : EnablePort
  Rectangular QAM Demodulator Baseband : commdigbbndam3/Rectangular QAM Demodulator Baseband  M=16  PowType=Min. distance between symbols  MinDist=2  AvgPow=1  PeakPow=1  Ph=0  Dec=Gray  Mapping=[0:15]  OutType=Bit  DecType=Hard decision  VarSource=Dialog  Variance=1  outDtype1=boolean  outDtype2=Inherit via internal rule  derotateFactorWordLen=16  denormFactorWordLen=16  prodOutWordLen=32  prodOutRoundingMode=Convergent  prodOutOverflowMode=Saturate  sumWordLen=32
  Out1 : Outport
  wires:
  Rectangular QAM Demodulator Baseband/1 -> Out1/1
  In1/1 -> Rectangular QAM Demodulator Baseband/1

== system Basic_DMT/IFFTaPIS/Create_Frame_for_IFFT/OFDMorDMT ==
  note: 1) Add Subsystem or Model blocks as valid variant choices.
      | 2) You cannot connect blocks at this level. At simulation, connectivity is automatically
      | determined, based on the active variant and port name matching.
  Sub1 : Inport
  Sub2 : Inport  Port=2
  Sub3 : Inport  Port=3
  Sub4 : Inport  Port=4
  Sub5 : Inport  Port=5
  Sub6 : Inport  Port=6
  Sub7 : Inport  Port=7
  Sub8 : Inport  Port=8
  Sub9 : Inport  Port=9
  Sub10 : Inport  Port=10
  Sub11 : Inport  Port=11
  Sub12 : Inport  Port=12
  Sub13 : Inport  Port=13
  Sub14 : Inport  Port=14
  Frame_DMT : Subsystem  VariantControl=dmtOfdm==2&&impulseResponse~=2
  Frame_OFDM : Subsystem  VariantControl=dmtOfdm==1&&impulseResponse~=2
  ImpulseResponse : Subsystem  VariantControl=impulseResponse==2
  Out1 : Outport

== system Basic_DMT/IFFTaPIS/Guard_Interval/None ==
  In1 : Inport
  Data Store Memory1 : DataStoreMemory  DataStoreName=k  OutDataTypeStr=double
  MATLAB Function : MATLAB Function  TreatAsAtomicUnit=on  SystemSampleTime=SystemPeriod*bitPerSymb*usedSubCar/fftLenActive
  Unbuffer1 : Unbuffer  SampleBasedProcessing=Same as frame based
  Out1 : Outport
  pop : Outport  Port=2
  wires:
  In1/1 -> Unbuffer1/1
  Unbuffer1/1 -> Out1/1
  MATLAB Function/1(push_en) -> pop/1
